simulink model "simulationStatePos"  (R2024a)
settings: Solver=VariableStepAuto  StartTime=0.0  StopTime=160  FixedStep=controlRate  RelTol=1e-3
InitFcn:
  | g = 9.81; %m/s^2
  | measRate = 0.001;
  | r = 0.03; % wheel radius
  | h = 0.1; % sensor 10cm above motor axel
  | 
  | noisePowerGyro = 0.0001;
  | noisePowerAccel = 0.0002;
  | noisePowerEnc = 0.0001;
  | 
  | % Bus object: encBus
  | clear elems;
  | elems(1) = Simulink.BusElement;
  | elems(1).Name = 'enc_count';
  | elems(1).Dimensions = 1;
  | elems(1).DimensionsMode = 'Fixed';
  | elems(1).DataType = 'int32';
  | elems(1).Complexity = 'real';
  | elems(1).Min = [];
  | elems(1).Max = [];
  | elems(1).DocUnits = '';
  | elems(1).Description = '';
  | 
  | elems(2) = Simulink.BusElement;
  | elems(2).Name = 'enc_dir';
  | elems(2).Dimensions = 1;
  | elems(2).DimensionsMode = 'Fixed';
  | elems(2).DataType = 'int8';
  | elems(2).Complexity = 'real';
  | elems(2).Min = [];
  | elems(2).Max = [];
  | elems(2).DocUnits = '';
  | elems(2).Description = '';
  | 
  | encBus = Simulink.Bus;
  | encBus.HeaderFile = '';
  | encBus.Description = '';
  | encBus.DataScope = 'Auto';
  | encBus.Alignment = -1;
  | encBus.PreserveElementDimensions = 0;
  | encBus.Elements = elems;
  | clear elems;
  | assignin('base','encBus', encBus);
undefined symbols (not defined in the file): ABPhase, accelToUnit, gearReductionRatio, gyroToUnit, PPR
settings Model: DataDictionary=globalData.sldd  VariantConfigurationObject=RobotVariantConfig  STM32="{\"PWMOutput\":[{\"ID\":\"sensorFusionWithControlTB66State:205\"},{\"ID\":\"sensorFusionWithControlTB66State:189\"},{\"ID\":\"sensorFusionWithControlTB66StatePos:2012\"},{\"ID\":\"sensorFusionWithControlTB66StatePos:2013\"}],\"DigitalPortWrite\":[{\"ID\":\"sensorFusionWithControlTB66State:1189\"},{\"ID\":\"sensorFusionWithControlTB66State:1225:7\"},{\"ID\":\"sensorFusionWithControlTB66State:1225:8\"},{\"ID\":\"sensorFusionWithControlTB66State:1225:9\"},{\"ID\":\"sensorFusionWithControlTB66State:1225:10\"},{\"ID\":\"sensorFusionWithControlTB66StatePos:1992\"},{\"ID\":\"sensorFusionWithControlTB66StatePos:2051:7\"},{\"ID\":\"sensorFusionWithControlTB66StatePos:2051:8\"},{\"ID\":\"sensorFusionWithControlTB66StatePos:2051:9\"},{\"ID\":\"sensorFusionWithControlTB66StatePos:2051:10\"}],\"EncoderBlock\":[{\"ID\":\"sensorFusionWithControlTB66State:1254\"},{\"ID\":\"sensorFusionWithControlTB66State:1257\"},{\"ID\":\"sensorFusionWithControlTB66StatePos:1993\"},{\"ID\":\"sensorFusionWithControlTB66StatePos:1994\"}],\"I2CControllerRead\":[{\"ID\":\"sensorFusionWithControlTB66State:1237:7\"},{\"ID\":\"sensorFusionWithControlTB66State:1237:18\"},{\"ID\":\"sensorFusionWithControlTB66State:1237:19\"},{\"ID\":\"sensorFusionWithControlTB66State:1237:20\"},{\"ID\":\"sensorFusionWithControlTB66State:1238:7\"},{\"ID\":\"sensorFusionWithControlTB66State:1238:15\"},{\"ID\":\"sensorFusionWithControlTB66State:1238:16\"},{\"ID\":\"sensorFusionWithControlTB66State:1238:17\"},{\"ID\":\"sensorFusionWithControlTB66StatePos:1237:18\"},{\"ID\":\"sensorFusionWithControlTB66StatePos:1237:19\"},{\"ID\":\"sensorFusionWithControlTB66StatePos:1237:20\"},{\"ID\":\"sensorFusionWithControlTB66StatePos:1238:7\"},{\"ID\":\"sensorFusionWithControlTB66StatePos:1238:15\"},{\"ID\":\"sensorFusionWithControlTB66StatePos:1238:16\"},{\"ID\":\"sensorFusionWithControlTB66StatePos:1238:17\"},{\"ID\":\"sensorFusionWithControlTB66StatePos:2053:7\"},{\"ID\":\"sensorFusionWithControlTB66StatePos:2053:18\"},{\"ID\":\"sensorFusionWithControlTB66StatePos:2053:19\"},{\"ID\":\"sensorFusionWithControlTB66StatePos:2053:20\"},{\"ID\":\"sensorFusionWithControlTB66StatePos:2054:7\"},{\"ID\":\"sensorFusionWithControlTB66StatePos:2054:15\"},{\"ID\":\"sensorFusionWithControlTB66StatePos:2054:16\"},{\"ID\":\"sensorFusionWithControlTB66StatePos:2054:17\"}],\"I2CControllerWrite\":[{\"ID\":\"sensorFusionWithControlTB66State:1237:21\"},{\"ID\":\"sensorFusionWithControlTB66State:1237:22\"},{\"ID\":\"sensorFusionWithControlTB66State:1237:23\"},{\"ID\":\"sensorFusionWithControlTB66State:1238:18\"},{\"ID\":\"sensorFusionWithControlTB66State:1238:19\"},{\"ID\":\"sensorFusionWithControlTB66State:1238:20\"},{\"ID\":\"sensorFusionWithControlTB66StatePos:1237:21\"},{\"ID\":\"sensorFusionWithControlTB66StatePos:1237:22\"},{\"ID\":\"sensorFusionWithControlTB66StatePos:1237:23\"},{\"ID\":\"sensorFusionWithControlTB66StatePos:1238:18\"},{\"ID\":\"sensorFusionWithControlTB66StatePos:1238:19\"},{\"ID\":\"sensorFusionWithControlTB66StatePos:1238:20\"},{\"ID\":\"sensorFusionWithControlTB66StatePos:2053:21\"},{\"ID\":\"sensorFusionWithControlTB66StatePos:2053:22\"},{\"ID\":\"sensorFusionWithControlTB66StatePos:2053:23\"},{\"ID\":\"sensorFusionWithControlTB66StatePos:2054:18\"},{\"ID\":\"sensorFusionWithControlTB66StatePos:2054:19\"},{\"ID\":\"sensorFusionWithControlTB66StatePos:2054:20\"}]}"  Creator=Peter  LastModifiedBy=Peter
settings OptimizationCC: DefaultParameterBehavior=Inlined  OptimizeBlockIOStorage=off  BufferReuse=off  ReuseModelBlockBuffer=off  GlobalBufferReuse=off  ExpressionFolding=off  EnableMemcpy=off  PassReuseOutputArgsAs=Individual arguments  LocalBlockOutputs=off  ZeroExternalMemoryAtStartup=off  ZeroInternalMemoryAtStartup=off  MaxStackSize=64  OptimizeDataStoreBuffers=off  BusAssignmentInplaceUpdate=off  OptimizationLevel=level0  OptimizationCustomize=off  EfficientTunableParamExpr=on
settings DebuggingCC: ParameterTunabilityLossMsg=error
settings HardwareCC: ProdBitPerPointer=32  ProdBitPerSizeT=32  ProdBitPerPtrDiffT=32  ProdLargestAtomicInteger=Long  ProdLargestAtomicFloat=Double  ProdWordSize=32  ProdLongLongMode=on  ProdHWDeviceType=ARM Compatible->ARM Cortex-M
settings SFSimCC: MATLABDynamicMemAlloc=off
settings RTWCC: Description=Embedded Coder  SystemTargetFile=ert.tlc  GenCodeOnly=on  TemplateMakefile=ert_default_tmf  Toolchain=GNU Tools for ARM Embedded Processors
settings CodeAppCC: GenerateComments=off  IgnoreCustomStorageClasses=off  OperatorAnnotations=on  SimulinkDataObjDesc=on  SFDataObjDesc=on  SimulinkBlockComments=off
settings ERTTargetCC: TargetLangStandard=C99 (ISO)  CodeReplacementLibrary=ARM Cortex-M  SupportComplex=off  ExtMode=on  ExtModeTransport=3  ExtModeStaticAlloc=on  ExtModeStaticAllocSize=2048  ExtModeMexFile=ext_xcp  ExtModeMexArgs=1 'COM11' 115200  ExtModeIntrfLevel=Level2 - Open  ERTCustomFileTemplate=example_file_process.tlc

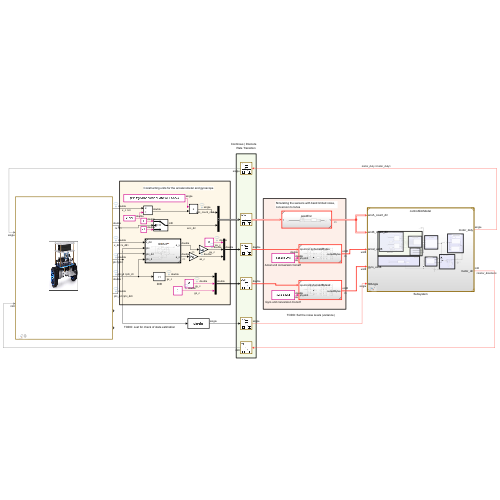
[thumbnail: Simulink's stored preview of the top-level diagram]
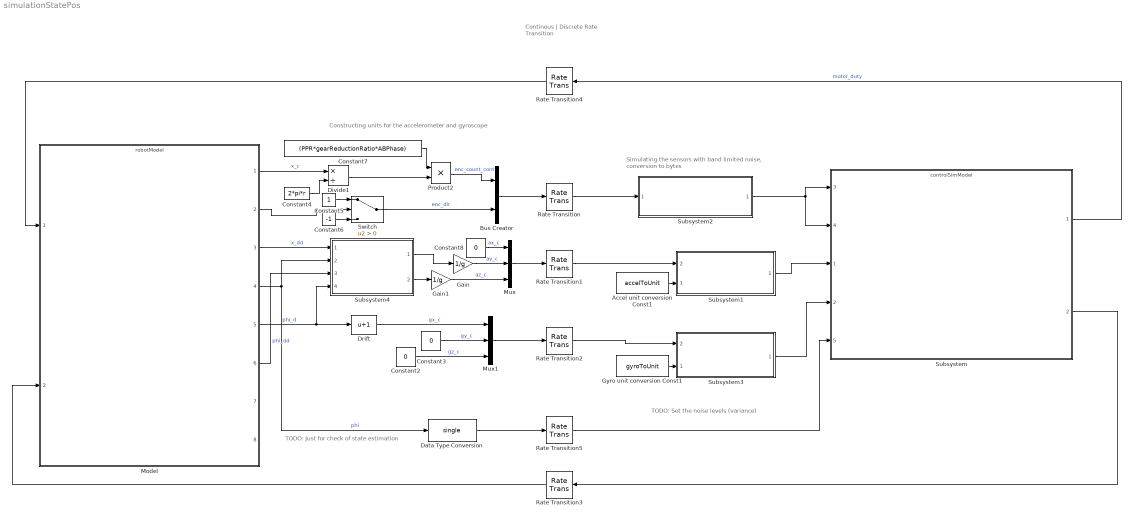
== system simulationStatePos ==
  note: TODO: Set the noise levels (variance)
  note: Continous | Discrete
      | 	Rate Transition
  note: Constructing units for the accelerometer and gyroscope
  note: Simulating the sensors with band limited noise, conversion to bytes
  note: TODO: Just for check of state estimation
  Accel unit conversion Const1 : Constant  Value=accelToUnit  OutDataTypeStr=double
  Bus Creator : BusCreator  Inputs=2
  Constant2 : Constant  Value=0
  Constant3 : Constant  Value=0
  Constant4 : Constant  Value=2*pi*r  OutDataTypeStr=double
  Constant5 : Constant
  Constant6 : Constant  Value=-1
  Constant7 : Constant  Value=(PPR*gearReductionRatio*ABPhase)  OutDataTypeStr=single
  Constant8 : Constant  Value=0
  Data Type Conversion : DataTypeConversion  OutDataTypeStr=single  SaturateOnIntegerOverflow=off  RndMeth=Floor
  Divide1 : Product  Inputs=*/
  Drift : Bias  Bias=1  SaturateOnIntegerOverflow=off
  Gain : Gain  Gain=1/g
  Gain1 : Gain  Gain=1/g
  Gyro unit conversion Const1 : Constant  Value=gyroToUnit  OutDataTypeStr=double
  Model : ModelReference  ModelNameDialog=robotModel.slx  SimulationMode=Normal  ModelReferenceVersion=1.12
      mask Display: image('documents/robotPic.png');
  Mux : Mux  Inputs=3
  Mux1 : Mux  Inputs=3
  Product2 : Product  OutDataTypeStr=single
  Rate Transition{,1..5} (6 alike) : RateTransition
  Subsystem : ModelReference  ModelNameDialog=controlSimModel.slx  SimulationMode=Normal  ModelReferenceVersion=1.201
      settings: PortSchema="{\"entries\":[{\"content\":{\"sides\":[{\"content\":{\"connectorIds\":[\"In3\",\"In4\",\"In1\",\"In2\",\"In5\"]},\"type\":\"ConnectorPlacement.EquallySpacedRectSide\",\"uuid\":\"607e8bf7-67b3-4598-837f-e1463bd54f31\"},{\"content\":{\"connectorIds\":[\"Out1\",\"Out2\"],\"side\":\"RIGHT\"},\"type\":\"ConnectorPlacement.EquallySpacedRectSide\",\"uuid\":\"665be0c9-ab78-4746-ae34-3e0e6aa01037\"},{\"content\":{\"side\":\"TOP\"},\"type\":\"ConnectorPlacement.EquallySpacedRectSide\",\"uuid\":\"2f225f8c-f7c2-494b-81d5-28791c2d479a\"}]},\"type\":\"ConnectorPlacement.EquallySpacedConnector\",\"uuid\":\"825e99fd-a980-4fe0-9e0d-c7ef55d58776\"}],\"packageUris\":[\"http://schema.mathworks.com/mf0/Connector/R2020b\"],\"version\":\"1.0\"}"
  Subsystem1 : Subsystem  TreatAsAtomicUnit=on  SystemSampleTime=measRate  ReferencedSubsystem=pyhscial2Bytes
      settings: PortSchema="{\"entries\":[{\"content\":{\"sides\":[{\"content\":{\"connectorIds\":[\"In2\",\"In1\"]},\"type\":\"ConnectorPlacement.EquallySpacedRectSide\",\"uuid\":\"53e2d529-3b42-4e12-904b-785035c56870\"},{\"content\":{\"connectorIds\":[\"Out1\"],\"side\":\"RIGHT\"},\"type\":\"ConnectorPlacement.EquallySpacedRectSide\",\"uuid\":\"e6f75a0f-b509-40fd-b19c-8042a83c0820\"},{\"content\":{\"side\":\"TOP\"},\"type\":\"ConnectorPlacement.EquallySpacedRectSide\",\"uuid\":\"82b0f229-96e7-4a10-a940-2f5032645be2\"}]},\"type\":\"ConnectorPlacement.EquallySpacedConnector\",\"uuid\":\"739ad422-8c2b-4e5b-9d03-011657a4e766\"}],\"packageUris\":[\"http://schema.mathworks.com/mf0/Connector/R2020b\"],\"version\":\"1.0\"}"
  Subsystem2 : Subsystem  TreatAsAtomicUnit=on  SystemSampleTime=measRate  ReferencedSubsystem=pos2Enc
  Subsystem3 : Subsystem  TreatAsAtomicUnit=on  SystemSampleTime=measRate  ReferencedSubsystem=pyhscial2Bytes2
      settings: PortSchema="{\"entries\":[{\"content\":{\"sides\":[{\"content\":{\"connectorIds\":[\"In2\",\"In1\"]},\"type\":\"ConnectorPlacement.EquallySpacedRectSide\",\"uuid\":\"53e2d529-3b42-4e12-904b-785035c56870\"},{\"content\":{\"connectorIds\":[\"Out1\"],\"side\":\"RIGHT\"},\"type\":\"ConnectorPlacement.EquallySpacedRectSide\",\"uuid\":\"e6f75a0f-b509-40fd-b19c-8042a83c0820\"},{\"content\":{\"side\":\"TOP\"},\"type\":\"ConnectorPlacement.EquallySpacedRectSide\",\"uuid\":\"82b0f229-96e7-4a10-a940-2f5032645be2\"}]},\"type\":\"ConnectorPlacement.EquallySpacedConnector\",\"uuid\":\"739ad422-8c2b-4e5b-9d03-011657a4e766\"}],\"packageUris\":[\"http://schema.mathworks.com/mf0/Connector/R2020b\"],\"version\":\"1.0\"}"
  Subsystem4 : Subsystem  TreatAsAtomicUnit=on  ReferencedSubsystem=tilt2Acc
  Switch : Switch  Criteria=u2 > Threshold  OutDataTypeStr=int8  SaturateOnIntegerOverflow=off  InputSameDT=off
  wires:
  Subsystem/1 -> Rate Transition4/1  "motor_duty"
  Subsystem/2 -> Rate Transition3/1
  Model/4 -> Data Type Conversion/1, Subsystem4/2  "phi"
  Model/5 -> Drift/1, Subsystem4/4  "phi_d"
  Constant2/1 -> Mux1/3  "gz_c"
  Constant3/1 -> Mux1/2  "gy_c"
  Constant4/1 -> Divide1/2
  Model/1 -> Divide1/1  "x_c"
  Divide1/1 -> Product2/2
  Constant7/1 -> Product2/1
  Model/2 -> Switch/2
  Constant5/1 -> Switch/1
  Constant6/1 -> Switch/3
  Switch/1 -> Bus Creator/2  "enc_dir"
  Mux1/1 -> Rate Transition2/1
  Product2/1 -> Bus Creator/1  "enc_count_cont"
  Bus Creator/1 -> Rate Transition/1
  Subsystem1/1 -> Subsystem/1
  Subsystem3/1 -> Subsystem/2
  Rate Transition3/1 -> Model/2
  Rate Transition4/1 -> Model/1
  Rate Transition1/1 -> Subsystem1/2
  Rate Transition2/1 -> Subsystem3/2
  Subsystem2/1 -> Subsystem/3, Subsystem/4
  Rate Transition/1 -> Subsystem2/1
  Accel unit conversion Const1/1 -> Subsystem1/1
  Gyro unit conversion Const1/1 -> Subsystem3/1
  Rate Transition5/1 -> Subsystem/5
  Data Type Conversion/1 -> Rate Transition5/1
  Model/3 -> Subsystem4/1  "x_dd"
  Model/6 -> Subsystem4/3  "phi_dd"
  Subsystem4/1 -> Gain/1
  Subsystem4/2 -> Gain1/1
  Constant8/1 -> Mux/1  "ax_c"
  Mux/1 -> Rate Transition1/1
  Gain/1 -> Mux/2  "ay_c"
  Gain1/1 -> Mux/3  "az_c"
  Drift/1 -> Mux1/1  "gx_c"
